simulink model "inverter_pwm2"  (Simulink 10.0)
settings: Solver=ode45  StartTime=0.0  StopTime=0.8  RelTol=1e-3  EnableMultiTasking=on
StopFcn:
  | T= ScopeData.time;
  | V_DC= ScopeData.signals(1,1).values;
  | V_LL=ScopeData2.signals.values;
  | subplot(2,1,1);
  | plot(T,V_LL);title('Line to Line Voltage Vab','fontsize',16);xlabel('t');ylabel('V');grid on;
  | subplot(2,1,2);
  | plot(T,V_DC);title('DC link Voltage Vdc','fontsize',16);xlabel('t');ylabel('V');grid on;
undefined symbols (not defined in the file): Ts
libraries: powerlib x18, simulink x1
settings Model: Creator=sample  LastModifiedBy=bhisma
settings DataIOCC: LimitDataPoints=on  SignalLoggingSaveFormat=ModelDataLogs
settings OptimizationCC: ExpressionDepthLimit=2147483647
settings DebuggingCC: SolverPrmCheckMsg=warning  FcnCallInpInsideContextMsg=warning  StateNameClashWarn=warning
settings GRTTargetCC: GeneratePreprocessorConditionals=Disable all
settings ConfigComp: CovExternalEMLEnable=off
settings SimscapeCC: SimscapeNormalizeSystem=off

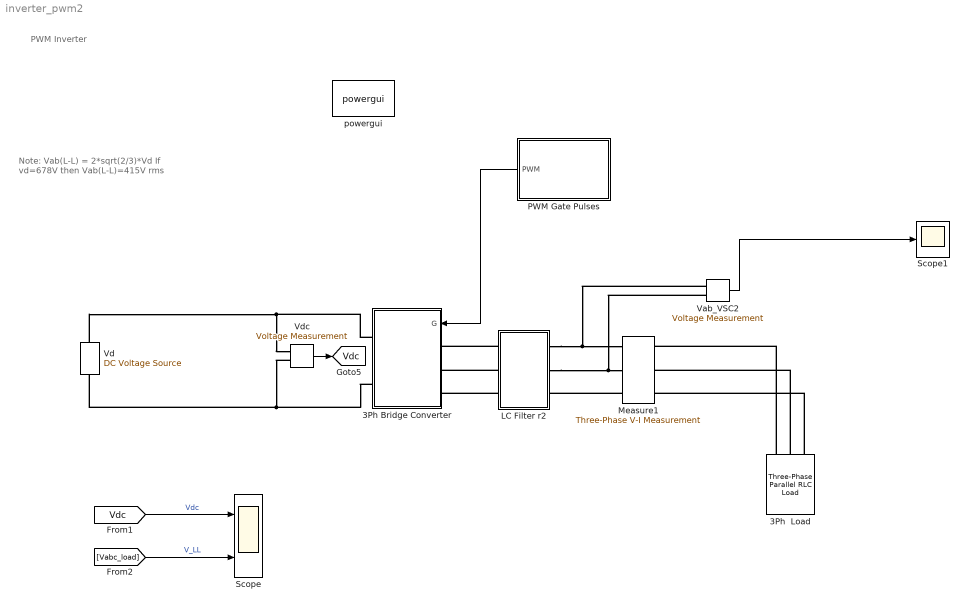
== system inverter_pwm2 ==
  note: PWM Inverter
  note: Note:
      | Vab(L-L) = 2*sqrt(2/3)*Vd
      | If vd=678V then  Vab(L-L)=415V rms
  "3Ph  Load " : powerlib/Elements/Three-Phase Parallel RLC Load  LConnTagsString=A|B|C  Configuration=Y (floating)  NominalVoltage=415  NominalFrequency=50  ActivePower=5e3  InductivePower=0  CapacitivePower=0  Measurements=None  LoadType=constant Z
      settings: SourceProductName=Simscape Electrical
  3Ph Bridge Converter : Subsystem
  LC Filter r2 : Subsystem  mask{L=10e-3, C=20e-6}
      mask prompts: L "Inductance"; C "Capacitance"
  Measure1 : powerlib/Measurements/Three-Phase V-I Measurement  VoltageMeasurement=phase-to-phase  SetLabelV=on  LabelV=Vabc_load  Vpu=off  VpuLL=off  CurrentMeasurement=no  SetLabelI=off  LabelI=I1  Ipu=off  Pbase=1e3  Vbase=380  OutputType=Magnitude  PhasorSimulation=off  PSBequivalent=0
      settings: SourceProductName=Simscape Electrical
  PWM Gate Pulses : Subsystem  mask{fc=50, fs=20000, m=1, inj=off, shift=0}
      mask prompts: fc "Control signal freq(Fc)"; fs "Swicting frequency"; m "Modulation Index"; inj "3rd harmonic Injection"; shift "Phase shift(Degrees)"
  Scope : Scope  NumInputPorts=2
  Scope1 : Scope
  Vab_VSC2 : powerlib/Measurements/Voltage Measurement  Tag=PoWeRsYsTeMmEaSuReMeNt  PhasorSimulation=off  OutputType=Magnitude  PSBequivalent=0
      settings: SourceProductName=Simscape Electrical
  Vd : powerlib/Electrical Sources/DC Voltage Source  Amplitude=415*2*sqrt(2/3)  Measurements=None
      settings: SourceProductName=Simscape Electrical
  "Vdc " : powerlib/Measurements/Voltage Measurement  Tag=PoWeRsYsTeMmEaSuReMeNt  PhasorSimulation=off  OutputType=Magnitude  PSBequivalent=0
      settings: SourceProductName=Simscape Electrical
  powergui : powerlib/powergui  Priority=1  SimulationMode=Continuous  SolverType=Tustin  SampleTime=50e-6  frequency=60  SPID=on  DisableSnubberDevices=off  DisableRonSwitches=off  DisableVfSwitches=off  SwTol=0  Interpol=off  DisplayEquations=off  FunctionMessages=off  frequencyindice=0  Pbase=100e6  ErrMax=1e-4  Iterations=50  UnitsV=kV  UnitsW=MW  echomessages=off  HookPort=off  EnableUseOfTLC=off  x0status=blocks  RestoreLinks=warning  ResistiveCurrentMeasurement=off  Ylog=off  Xlog=on  ShowGrid=off  save=off  variable=ZData  structure=ScopeData2  ZoomFFT=off  StartTime=0.6  cycles=4  DisplayStyle=4  fundamental=50  FreqAxis=on  MaxFrequency=650  frequencyindicesteady=1  display=off  methode=off
      settings: SourceProductName=Simscape Electrical
  tag scope: Vdc=global
  wires:
  "Vdc "/1 -> [Vdc]
  [Vabc_load] -> Scope/2  "V_LL"
  [Vdc] -> Scope/1  "Vdc"
  PWM Gate Pulses/1(PWM) -> 3Ph Bridge Converter/1(G)
  Vab_VSC2/1 -> Scope1/1
  connections:
  "3Ph  Load "/LConn1 -- Measure1/RConn1
  "3Ph  Load "/LConn2 -- Measure1/RConn2
  "Vdc "/LConn2 -- Vd/LConn1 -- 3Ph Bridge Converter/RConn2
  Vd/RConn1 -- "Vdc "/LConn1 -- 3Ph Bridge Converter/RConn1
  "3Ph  Load "/LConn3 -- Measure1/RConn3
  Vab_VSC2/LConn1 -- Measure1/LConn1 -- LC Filter r2/RConn1
  Vab_VSC2/LConn2 -- LC Filter r2/RConn2 -- Measure1/LConn2
  LC Filter r2/LConn1 -- 3Ph Bridge Converter/LConn1
  LC Filter r2/LConn2 -- 3Ph Bridge Converter/LConn2
  LC Filter r2/LConn3 -- 3Ph Bridge Converter/LConn3
  Measure1/LConn3 -- LC Filter r2/RConn3

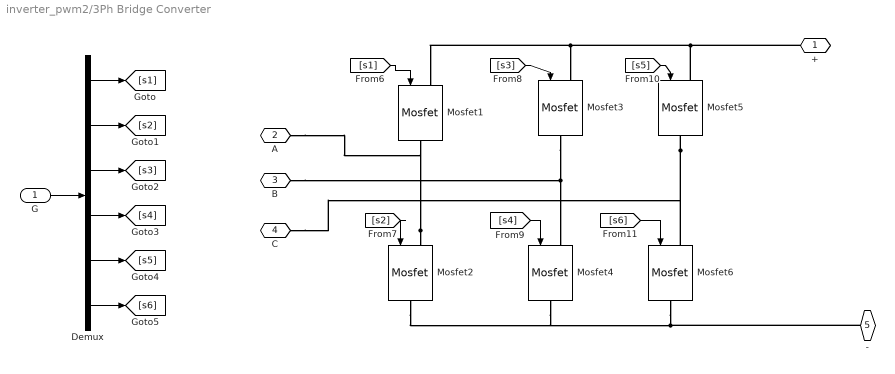
== system inverter_pwm2/3Ph Bridge Converter ==
  G : Inport
  Demux : Demux  Outputs=6
  Mosfet{1..6} (6 alike) : powerlib/Power Electronics/Mosfet  Ron=0.1  Lon=0  Rd=0.01  Vfd=0  IC=0  Rs=1e5  Cs=inf  Measurements=off
      settings: SourceProductName=Simscape Electrical
  + : PMIOPort  Side=Right
  A : PMIOPort  Port=2  Side=Left
  B : PMIOPort  Port=3  Side=Left
  C : PMIOPort  Port=4  Side=Left
  - : PMIOPort  Port=5  Side=Right
  wires:
  [s1] -> Mosfet1/1
  [s2] -> Mosfet2/1
  [s3] -> Mosfet3/1
  [s4] -> Mosfet4/1
  [s5] -> Mosfet5/1
  [s6] -> Mosfet6/1
  Demux/1 -> [s1]
  Demux/2 -> [s2]
  Demux/3 -> [s3]
  Demux/4 -> [s4]
  Demux/5 -> [s5]
  Demux/6 -> [s6]
  G/1 -> Demux/1
  connections:
  Mosfet5/LConn1 -- Mosfet1/LConn1 -- Mosfet3/LConn1 -- +/RConn1
  Mosfet6/RConn1 -- Mosfet2/RConn1 -- Mosfet4/RConn1 -- -/RConn1
  Mosfet2/LConn1 -- Mosfet1/RConn1 -- A/RConn1
  Mosfet3/RConn1 -- Mosfet4/LConn1 -- B/RConn1
  Mosfet5/RConn1 -- Mosfet6/LConn1 -- C/RConn1

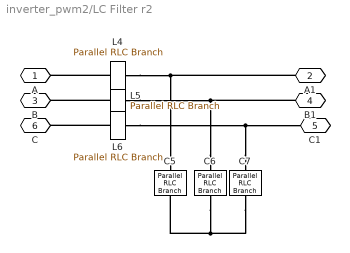
== system inverter_pwm2/LC Filter r2 ==
  C5 : powerlib/Elements/Parallel RLC Branch  LConnTagsString=a  RConnTagsString=__new0  BranchType=C  Resistance=inf  Inductance=inf  SetiL0=off  InitialCurrent=0  Capacitance=C  Setx0=off  InitialVoltage=0  Measurements=None
      settings: SourceProductName=Simscape Electrical
  C6 : powerlib/Elements/Parallel RLC Branch  LConnTagsString=a  RConnTagsString=__new0  BranchType=C  Resistance=inf  Inductance=inf  SetiL0=off  InitialCurrent=0  Capacitance=C  Setx0=off  InitialVoltage=0  Measurements=None
      settings: SourceProductName=Simscape Electrical
  C7 : powerlib/Elements/Parallel RLC Branch  LConnTagsString=a  RConnTagsString=__new0  BranchType=C  Resistance=inf  Inductance=inf  SetiL0=off  InitialCurrent=0  Capacitance=C  Setx0=off  InitialVoltage=0  Measurements=None
      settings: SourceProductName=Simscape Electrical
  L4 : powerlib/Elements/Parallel RLC Branch  LConnTagsString=a  RConnTagsString=__new0  BranchType=L  Resistance=inf  Inductance=L  SetiL0=off  InitialCurrent=0  Capacitance=1.3e-3  Setx0=off  InitialVoltage=0  Measurements=None
      settings: SourceProductName=Simscape Electrical
  L5 : powerlib/Elements/Parallel RLC Branch  LConnTagsString=a  RConnTagsString=__new0  BranchType=L  Resistance=inf  Inductance=L  SetiL0=off  InitialCurrent=0  Capacitance=1.3e-3  Setx0=off  InitialVoltage=0  Measurements=None
      settings: SourceProductName=Simscape Electrical
  L6 : powerlib/Elements/Parallel RLC Branch  LConnTagsString=a  RConnTagsString=__new0  BranchType=L  Resistance=inf  Inductance=L  SetiL0=off  InitialCurrent=0  Capacitance=1.3e-3  Setx0=off  InitialVoltage=0  Measurements=None
      settings: SourceProductName=Simscape Electrical
  A : PMIOPort  Side=Left
  A1 : PMIOPort  Port=2  Side=Right
  B : PMIOPort  Port=3  Side=Left
  B1 : PMIOPort  Port=4  Side=Right
  C1 : PMIOPort  Port=5  Side=Right
  C : PMIOPort  Port=6  Side=Left
  connections:
  L4/LConn1 -- A/RConn1
  L6/LConn1 -- C/RConn1
  C5/RConn1 -- C7/RConn1 -- C6/RConn1
  L5/LConn1 -- B/RConn1
  C6/LConn1 -- B1/RConn1 -- L5/RConn1
  L4/RConn1 -- A1/RConn1 -- C5/LConn1
  C7/LConn1 -- C1/RConn1 -- L6/RConn1

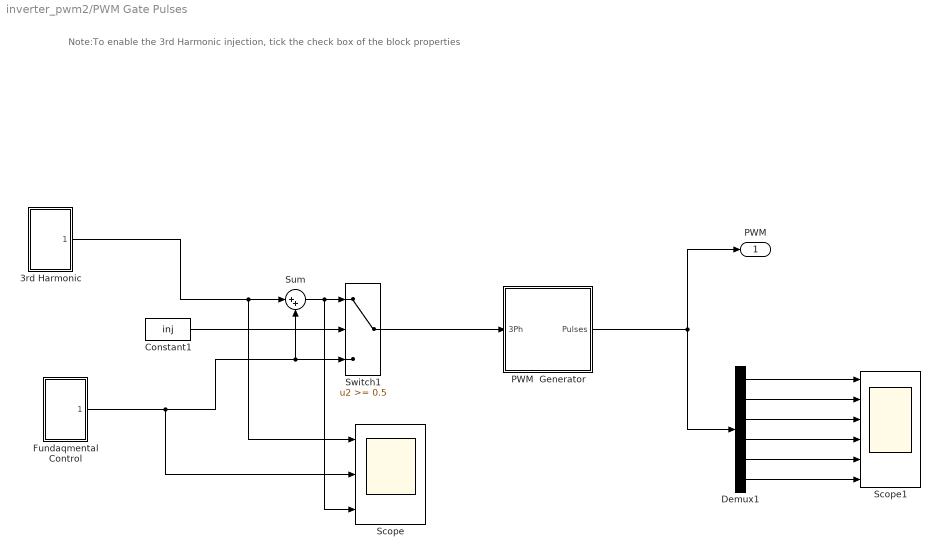
== system inverter_pwm2/PWM Gate Pulses ==
  note: Note:To enable the 3rd Harmonic injection, tick the check box of the block properties
  3rd Harmonic : Subsystem
  Constant1 : Constant  Value=inj  SampleTime=Ts
  Demux1 : Demux  Outputs=6
  Fundaqmental Control : Subsystem
  PWM  Generator : Subsystem  InitFcn=Ts=2e-6
  Scope : Scope  NumInputPorts=3
  Scope1 : Scope  NumInputPorts=6
  Sum : Sum  Inputs=|++
  Switch1 : Switch  Threshold=0.5  SampleTime=Ts  SaturateOnIntegerOverflow=on  InputSameDT=on
  PWM : Outport
  wires:
  Demux1/1 -> Scope1/1
  Demux1/2 -> Scope1/2
  Demux1/3 -> Scope1/3
  Demux1/4 -> Scope1/4
  Demux1/5 -> Scope1/5
  Demux1/6 -> Scope1/6
  PWM  Generator/1(Pulses) -> PWM/1, Demux1/1
  Constant1/1 -> Switch1/2
  Switch1/1 -> PWM  Generator/1(3Ph)
  Sum/1 -> Scope/3, Switch1/1
  3rd Harmonic/1(Sin(3wt)) -> Scope/1, Sum/1
  Fundaqmental Control/1(Sin(wt)) -> Scope/2, Sum/2, Switch1/3

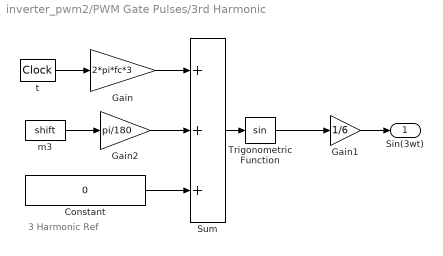
== system inverter_pwm2/PWM Gate Pulses/3rd Harmonic ==
  note: 3 Harmonic Ref
  Constant : Constant  Value=0  SampleTime=Ts
  Gain : Gain  Gain=2*pi*fc*3  SaturateOnIntegerOverflow=on  OutDataTypeStr=Inherit: Same as input  ParamDataTypeStr=Inherit: Same as input
  Gain1 : Gain  Gain=1/6
  Gain2 : Gain  Gain=pi/180  SaturateOnIntegerOverflow=on  OutDataTypeStr=Inherit: Same as input  ParamDataTypeStr=Inherit: Same as input
  Sum : Sum  Inputs=+++  SampleTime=Ts  SaturateOnIntegerOverflow=on  InputSameDT=on  OutDataTypeStr=Inherit: Same as first input
  Trigonometric Function : Trigonometry  SampleTime=Ts
  m3 : Constant  Value=shift  SampleTime=Ts
  t : DigitalClock  SampleTime=Ts
  Sin(3wt) : Outport
  wires:
  t/1 -> Gain/1
  Gain/1 -> Sum/1
  Gain2/1 -> Sum/2
  m3/1 -> Gain2/1
  Constant/1 -> Sum/3
  Sum/1 -> Trigonometric Function/1
  Trigonometric Function/1 -> Gain1/1
  Gain1/1 -> Sin(3wt)/1

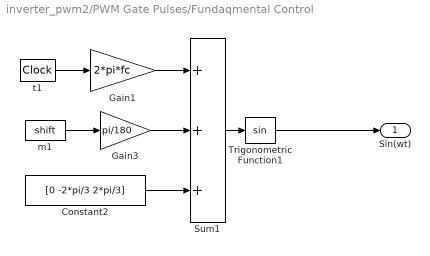
== system inverter_pwm2/PWM Gate Pulses/Fundaqmental Control ==
  Constant2 : Constant  Value=[0 -2*pi/3 2*pi/3]  SampleTime=Ts
  Gain1 : Gain  Gain=2*pi*fc  SaturateOnIntegerOverflow=on  OutDataTypeStr=Inherit: Same as input  ParamDataTypeStr=Inherit: Same as input
  Gain3 : Gain  Gain=pi/180  SaturateOnIntegerOverflow=on  OutDataTypeStr=Inherit: Same as input  ParamDataTypeStr=Inherit: Same as input
  Sum1 : Sum  Inputs=+++  SampleTime=Ts  SaturateOnIntegerOverflow=on  InputSameDT=on  OutDataTypeStr=Inherit: Same as first input
  Trigonometric Function1 : Trigonometry  SampleTime=Ts
  m1 : Constant  Value=shift  SampleTime=Ts
  t1 : DigitalClock  SampleTime=Ts
  Sin(wt) : Outport
  wires:
  Trigonometric Function1/1 -> Sin(wt)/1
  t1/1 -> Gain1/1
  Gain1/1 -> Sum1/1
  Gain3/1 -> Sum1/2
  m1/1 -> Gain3/1
  Constant2/1 -> Sum1/3
  Sum1/1 -> Trigonometric Function1/1

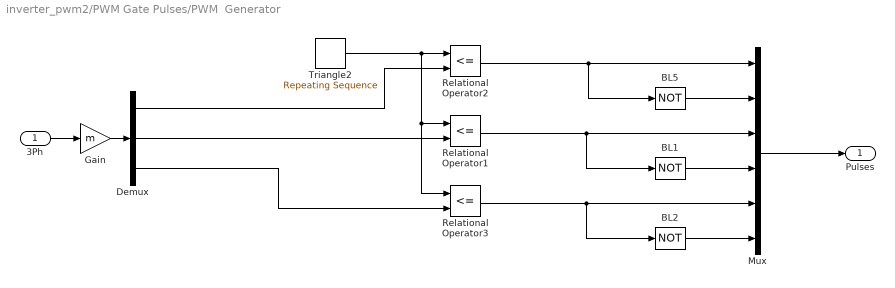
== system inverter_pwm2/PWM Gate Pulses/PWM  Generator ==
  3Ph : Inport
  BL1 : Logic  Operator=NOT  Inputs=1  SampleTime=Ts
  BL2 : Logic  Operator=NOT  Inputs=1  SampleTime=Ts
  BL5 : Logic  Operator=NOT  Inputs=1  SampleTime=Ts
  Demux : Demux  Outputs=3
  Gain : Gain  Gain=m
  Mux : Mux  Inputs=6
  Relational Operator1 : RelationalOperator  Operator=<=  RndMeth=Nearest
  Relational Operator2 : RelationalOperator  Operator=<=  RndMeth=Nearest
  Relational Operator3 : RelationalOperator  Operator=<=  RndMeth=Nearest
  Triangle2 : simulink/Sources/Repeating Sequence  rep_seq_t=[0 1/fs/4 3/fs/4 1/fs]  rep_seq_y=[0 -1 1 0]
  Pulses : Outport
  wires:
  Mux/1 -> Pulses/1
  Relational Operator2/1 -> Mux/1, BL5/1
  BL5/1 -> Mux/2
  Relational Operator1/1 -> BL1/1, Mux/3
  Demux/1 -> Relational Operator2/2
  Triangle2/1 -> Relational Operator3/1, Relational Operator1/1, Relational Operator2/1
  BL1/1 -> Mux/4
  Relational Operator3/1 -> BL2/1, Mux/5
  BL2/1 -> Mux/6
  Demux/3 -> Relational Operator3/2
  Demux/2 -> Relational Operator1/2
  3Ph/1 -> Gain/1
  Gain/1 -> Demux/1
